simulink model "MixingTank_NonlinearModel_Simulink2019b"  (R2019b)
settings: Solver=ode4  StartTime=0.0  StopTime=SIM_TIME  FixedStep=STEP_SIZE  RelTol=1e-3
undefined symbols (not defined in the file): At, Cv, kh, kt, kv, x0
settings Model: Creator=Roberto  LastModifiedBy=roga
settings DataIOCC: ReturnWorkspaceOutputs=off
settings DebuggingCC: ArithmeticOperatorsInVariantConditions=warning
settings SFSimCC: SimUseLocalCustomCode=off  CustomCodeUndefinedFunction=UseInterfaceOnly
settings RTWCC: RTWUseLocalCustomCode=off

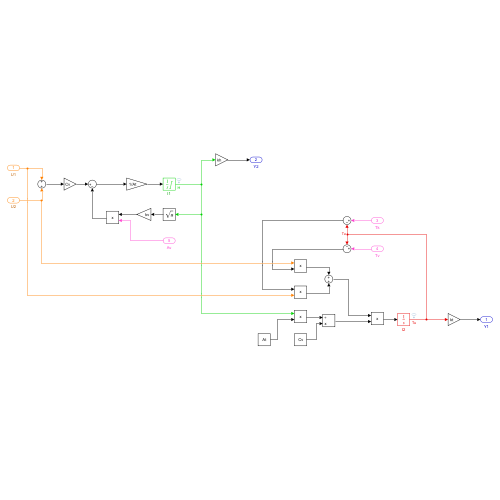
[thumbnail: Simulink's stored preview of the top-level diagram]
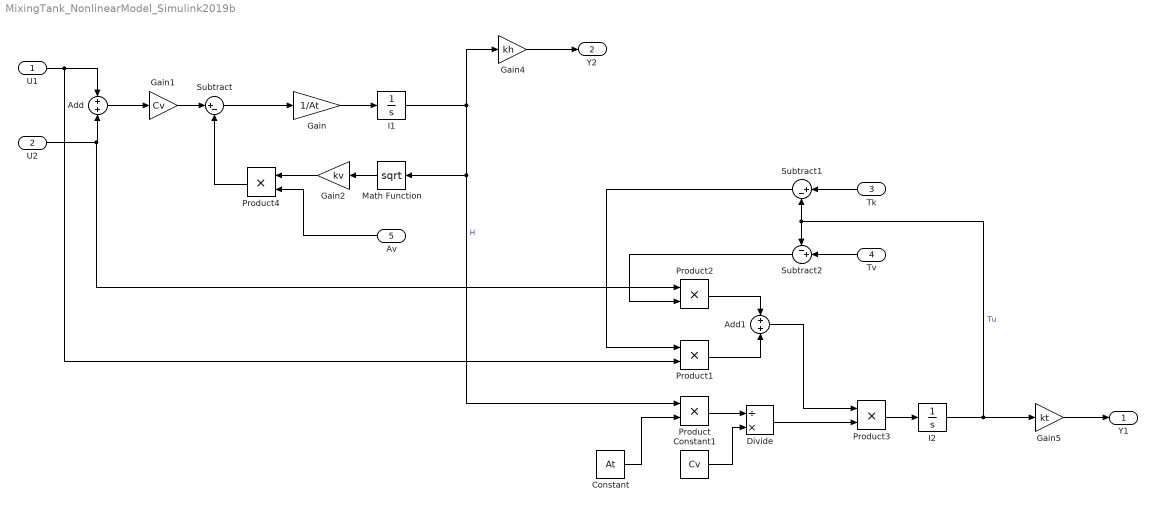
== system MixingTank_NonlinearModel_Simulink2019b ==
  U1 : Inport
  U2 : Inport  Port=2
  Tk : Inport  Port=3
  Tv : Inport  Port=4
  Av : Inport  Port=5
  Add : Sum
  Add1 : Sum
  Constant : Constant  Value=At
  Constant1 : Constant  Value=Cv
  Divide : Product  Inputs=/*
  Gain : Gain  Gain=1/At
  Gain1 : Gain  Gain=Cv
  Gain2 : Gain  Gain=kv
  Gain4 : Gain  Gain=kh
  Gain5 : Gain  Gain=kt
  I1 : Integrator  Priority=1  InitialCondition=x0(1)  LimitOutput=on  LowerSaturationLimit=0
  I2 : Integrator  Priority=2  InitialCondition=x0(2)
  Math Function : Math  Operator=sqrt  SignedPower=on  SaturateOnIntegerOverflow=on
  Product{,1..4} (5 alike) : Product  RndMeth=Zero
  Subtract : Sum  Inputs=|+-
  Subtract1 : Sum  Inputs=|+-
  Subtract2 : Sum  Inputs=-+|
  Y1 : Outport  VectorParamsAs1DForOutWhenUnconnected=off
  Y2 : Outport  Port=2  VectorParamsAs1DForOutWhenUnconnected=off
  wires:
  Math Function/1 -> Gain2/1
  Gain2/1 -> Product4/1
  Product/1 -> Divide/1
  Subtract1/1 -> Product1/1
  Product3/1 -> I2/1
  I1/1 -> Math Function/1, Product/1, Gain4/1  "H"
  Product4/1 -> Subtract/2
  Av/1 -> Product4/2
  Gain1/1 -> Subtract/1
  Add1/1 -> Product3/1
  Constant/1 -> Product/2
  Subtract2/1 -> Product2/2
  Tk/1 -> Subtract1/1
  Add/1 -> Gain1/1
  U1/1 -> Product1/2, Add/1
  Constant1/1 -> Divide/2
  Gain/1 -> I1/1
  U2/1 -> Product2/1, Add/2
  Subtract/1 -> Gain/1
  I2/1 -> Gain5/1, Subtract2/1, Subtract1/2  "Tu"
  Gain4/1 -> Y2/1
  Gain5/1 -> Y1/1
  Tv/1 -> Subtract2/2
  Divide/1 -> Product3/2
  Product2/1 -> Add1/1
  Product1/1 -> Add1/2
